simulink model "Assignment3_7"  (R2021a)
settings: Solver=VariableStepAuto  StartTime=0.0  StopTime=10.0  RelTol=1e-3
undefined symbols (not defined in the file): A1, B
settings Model: Creator=TITIR  LastModifiedBy=TITIR

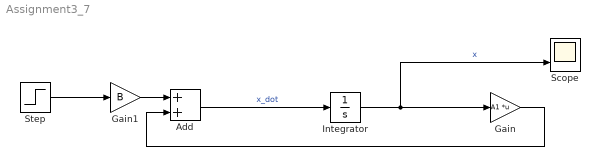
== system Assignment3_7 ==
  Add : Sum
  Gain : Gain  Gain=A1  Multiplication=Matrix(K*u)
  Gain1 : Gain  Gain=B
  Integrator : Integrator
  Scope : Scope  NumInputPorts=2
  Step : Step  SampleTime=0
  wires:
  Integrator/1 -> Scope/2, Gain/1  "x"
  Add/1 -> Integrator/1  "x_dot"
  Gain/1 -> Add/2
  Gain1/1 -> Add/1
  Step/1 -> Gain1/1
